simulink model "collide_between"  (R2018a)
settings: Solver=VariableStepAuto  StartTime=0.0  StopTime=120  FixedStep=0.01  MaxStep=.01  RelTol=1e-3
settings Model: Creator=U500304  LastModifiedBy=U500304
settings SolverCC: ZeroCrossAlgorithm=Adaptive
settings DataIOCC: SaveOutput=off  SaveTime=off
settings DebuggingCC: MaxConsecutiveZCsMsg=warning

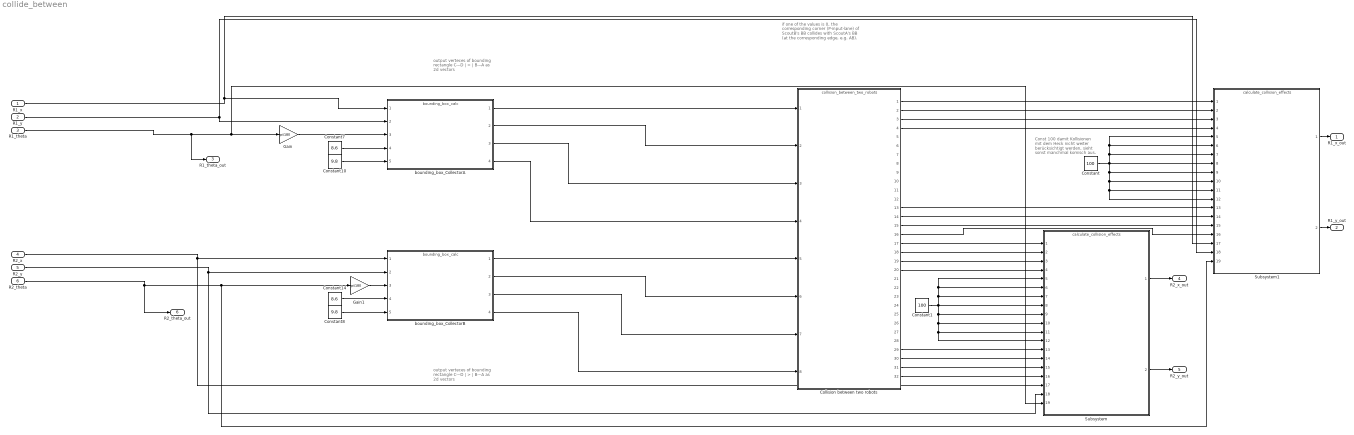
== system collide_between ==
  note: Const 100 damit Kollisionen
      | mit dem Heck nicht weiter
      | berücksichtigt werden, sieht sonst
      | manchmal komisch aus.
  note: if one of the values is 0, the corresponding corner (P-input-lane) of ScoutB's BB collides with ScoutA's BB (at the corresponding edge, e.g. AB).
  note: output verteces of
      | bounding rectangle
      | C---D
      | |  >  |
      | B---A  as 2d vectors
  note: output verteces of
      | bounding rectangle
      | C---D
      | |  >  |
      | B---A  as 2d vectors
  R1_x : Inport  OutDataTypeStr=double  PortDimensions=1  SampleTime=0
  R1_y : Inport  Port=2  OutDataTypeStr=double  PortDimensions=1  SampleTime=0
  R1_theta : Inport  Port=3  OutDataTypeStr=double  PortDimensions=1  SampleTime=0
  R2_x : Inport  Port=4  OutDataTypeStr=double  PortDimensions=1  SampleTime=0
  R2_y : Inport  Port=5  OutDataTypeStr=double  PortDimensions=1  SampleTime=0
  R2_theta : Inport  Port=6  OutDataTypeStr=double  PortDimensions=1  SampleTime=0
  Collision between two robots : ModelReference  ModelNameDialog=collision_between_two_robots  SimulationMode=Normal  ModelReferenceVersion=1.665
  Constant : Constant  Value=100
  Constant1 : Constant  Value=100
  Constant10 : Constant  Value=9.8
  Constant14 : Constant  Value=8.6
  Constant7 : Constant  Value=8.6
  Constant8 : Constant  Value=9.8
  Gain : Gain  Gain=pi/180
  Gain1 : Gain  Gain=pi/180
  Subsystem : ModelReference  ModelNameDialog=calculate_collision_effects  SimulationMode=Normal  ModelReferenceVersion=1.719
  Subsystem1 : ModelReference  ModelNameDialog=calculate_collision_effects  SimulationMode=Normal  ModelReferenceVersion=1.719
  bounding_box_CollectorA : ModelReference  ModelNameDialog=bounding_box_calc  SimulationMode=Normal  ModelReferenceVersion=1.661
  bounding_box_CollectorB : ModelReference  ModelNameDialog=bounding_box_calc  SimulationMode=Normal  ModelReferenceVersion=1.661
  R1_x_out : Outport  OutDataTypeStr=double  PortDimensions=1  SampleTime=0
  R1_y_out : Outport  Port=2  OutDataTypeStr=double  PortDimensions=1  SampleTime=0
  R1_theta_out : Outport  Port=3  OutDataTypeStr=double  PortDimensions=1  SampleTime=0
  R2_x_out : Outport  Port=4  OutDataTypeStr=double  PortDimensions=1  SampleTime=0
  R2_y_out : Outport  Port=5  OutDataTypeStr=double  PortDimensions=1  SampleTime=0
  R2_theta_out : Outport  Port=6  OutDataTypeStr=double  PortDimensions=1  SampleTime=0
  wires:
  Collision between two robots/13 -> Subsystem1/13
  Collision between two robots/17 -> Subsystem/1
  Collision between two robots/31 -> Subsystem/15
  Collision between two robots/3 -> Subsystem1/3
  R2_x/1 -> bounding_box_CollectorB/1, Subsystem/17
  bounding_box_CollectorB/1 -> Collision between two robots/5
  Collision between two robots/1 -> Subsystem1/1
  Collision between two robots/4 -> Subsystem1/4
  Collision between two robots/29 -> Subsystem/13
  Subsystem1/2 -> R1_y_out/1
  bounding_box_CollectorA/3 -> Collision between two robots/3
  R1_theta/1 -> R1_theta_out/1, Subsystem/19, Gain/1
  R2_theta/1 -> Gain1/1, Subsystem1/19, R2_theta_out/1
  Subsystem1/1 -> R1_x_out/1
  R1_x/1 -> bounding_box_CollectorA/1, Subsystem1/17
  bounding_box_CollectorA/1 -> Collision between two robots/1
  Collision between two robots/16 -> Subsystem1/16
  bounding_box_CollectorA/4 -> Collision between two robots/4
  Collision between two robots/20 -> Subsystem/4
  Collision between two robots/2 -> Subsystem1/2
  bounding_box_CollectorB/4 -> Collision between two robots/8
  R2_y/1 -> Subsystem/18, bounding_box_CollectorB/2
  Constant8/1 -> bounding_box_CollectorB/5
  R1_y/1 -> Subsystem1/18, bounding_box_CollectorA/2
  Collision between two robots/15 -> Subsystem1/15
  Gain/1 -> bounding_box_CollectorA/3
  Subsystem/2 -> R2_y_out/1
  Collision between two robots/14 -> Subsystem1/14
  Collision between two robots/32 -> Subsystem/16
  Constant10/1 -> bounding_box_CollectorA/5
  Gain1/1 -> bounding_box_CollectorB/3
  Constant7/1 -> bounding_box_CollectorA/4
  bounding_box_CollectorA/2 -> Collision between two robots/2
  Collision between two robots/18 -> Subsystem/2
  Collision between two robots/30 -> Subsystem/14
  bounding_box_CollectorB/3 -> Collision between two robots/7
  Constant14/1 -> bounding_box_CollectorB/4
  Subsystem/1 -> R2_x_out/1
  Collision between two robots/19 -> Subsystem/3
  bounding_box_CollectorB/2 -> Collision between two robots/6
  Constant/1 -> Subsystem1/8, Subsystem1/9, Subsystem1/10, Subsystem1/11, Subsystem1/12, Subsystem1/5, Subsystem1/6, Subsystem1/7
  Constant1/1 -> Subsystem/8, Subsystem/7, Subsystem/6, Subsystem/5, Subsystem/9, Subsystem/10, Subsystem/11, Subsystem/12
